simulink model "AddPoles"  (R2020a)
settings: Solver=VariableStepAuto  StartTime=0.0  StopTime=10.0  RelTol=1e-3
model workspace (MAT data in the model file):
  K = 2000
  Sig = Simulink.Signal
  Sig.DataType = 'auto'
  Sig.Dimensions = -1
  Sig.DimensionsMode = 'auto'
  Sig.Complexity = 'auto'
  Sig.SampleTime = -1
  Sig.SamplingMode = 'auto'
settings Model: Creator=Kimo Store  LastModifiedBy=Kimo Store

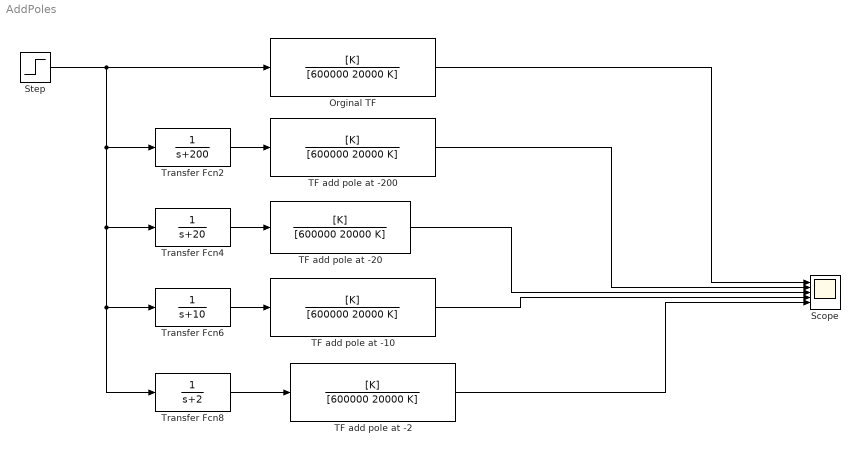
== system AddPoles ==
  Orginal TF : TransferFcn  Numerator=[K]  Denominator=[600000 20000 K]
  Scope : Scope  NumInputPorts=5
  Step : Step  Time=0  SampleTime=0
  TF add pole at -{2,10,20,200} (4 alike) : TransferFcn  Numerator=[K]  Denominator=[600000 20000 K]
  Transfer Fcn2 : TransferFcn  Denominator=[1 200]
  Transfer Fcn4 : TransferFcn  Denominator=[1 20]
  Transfer Fcn6 : TransferFcn  Denominator=[1 10]
  Transfer Fcn8 : TransferFcn  Denominator=[1 2]
  wires:
  Step/1 -> Orginal TF/1, Transfer Fcn8/1, Transfer Fcn6/1, Transfer Fcn4/1, Transfer Fcn2/1
  Orginal TF/1 -> Scope/1
  TF add pole at -200/1 -> Scope/2
  Transfer Fcn2/1 -> TF add pole at -200/1
  Transfer Fcn4/1 -> TF add pole at -20/1
  Transfer Fcn6/1 -> TF add pole at -10/1
  Transfer Fcn8/1 -> TF add pole at -2/1
  TF add pole at -20/1 -> Scope/3
  TF add pole at -10/1 -> Scope/4
  TF add pole at -2/1 -> Scope/5
